simulink model "backstepping"  (R2022b)
settings: Solver=ode45  StartTime=0.0  StopTime=20  RelTol=1e-5
settings Model: Creator=Alex  LastModifiedBy=Alex

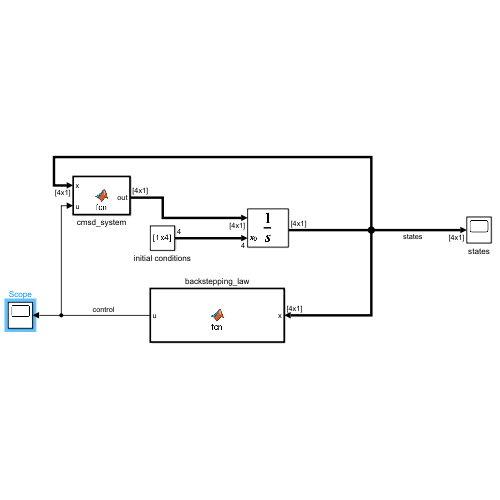
[thumbnail: Simulink's stored preview of the top-level diagram]
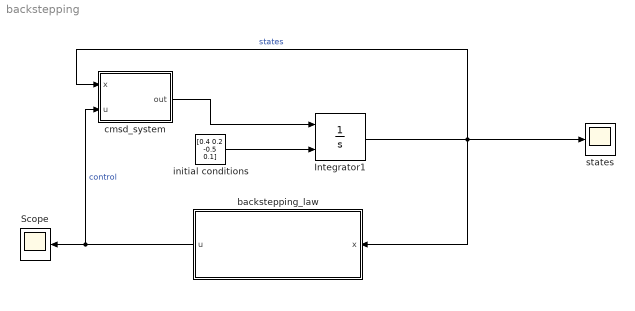
== system backstepping ==
  Integrator1 : Integrator  InitialConditionSource=external  InitialCondition=[0.1 0.02 -0.1 -0.1]'
  Scope : Scope
  backstepping_law : MATLAB Function  TreatAsAtomicUnit=on
  cmsd_system : MATLAB Function  TreatAsAtomicUnit=on
  initial conditions : Constant  Value=[0.4 0.2 -0.5 0.1]
  states : Scope
  wires:
  initial conditions/1 -> Integrator1/2
  cmsd_system/1(out) -> Integrator1/1
  Integrator1/1 -> states/1, cmsd_system/1(x), backstepping_law/1(x)  "states"
  backstepping_law/1(u) -> cmsd_system/2(u), Scope/1  "control"

== matlab function backstepping/backstepping_law ==
  data: x input; u output
function u = fcn(x)
k1=2/5; % N/m
k2=1;
m1=1; % kg
m2=2;
delta1=1/10; %
delta2=1/5;
miu1=1/6; %
miu2=1/10;

x1=x(1);
x2=x(2);
x3=x(3);
x4=x(4);

phi=3*x1^2*x3-3*x1*x2*x3+x2^2*x3-(1-k1-k2)*x1-k2*x3;
z=x(4)-phi;
k=3;
u=-m2*(x2-delta2/m2*x(4)-k2/m2*(x(2)-x(1))+miu2/m2*(x(2)-x(1))^3 ...
    -x3*(6*x1*x3-3*x2*x3+k1+k1-1) -x4*(-3*x1*x3+2*x2*x3)- ...
    (-delta1/m1*x(3)-k1/m1*x(1)+miu1/m1 * x(1)^3 - k2/m1 * (x(1)-x(2))+miu2/m1*(x(1)-x(2))^3)*(3*x1^2-3*x1*x2+x2^2-k2)+ ...
    k*z);

== matlab function backstepping/cmsd_system ==
  data: x input; u input; out output
function out = fcn(x,u)

k1=2/5; % N/m
k2=1;
m1=1; % kg
m2=2;
delta1=1/10; %Ns/m
delta2=1/5;
miu1=1/6; %
miu2=1/10;
g=[0 0 0 1/m2]';

xdot=[x(3);...
      x(4);...
      -delta1/m1*x(3)-k1/m1*x(1)+miu1/m1 * x(1)^3 - k2/m1 * (x(1)-x(2))+miu2/m1*(x(1)-x(2))^3;...
      -delta2/m2*x(4)-k2/m2*(x(2)-x(1))+miu2/m2*(x(2)-x(1))^3];



out= xdot+g*u;
